simulink model "Ex1Mdl"  (R2019b)
settings: Solver=VariableStepAuto  StartTime=0.0  StopTime=20  RelTol=1e-3
values from neighbouring files (symbols this model uses):
  k1 = p(4)    [Ex1.m]
  k2 = p(3)    [Ex1.m]
  k3 = p(2)    [Ex1.m]
  z0 = [0.001 0 0.2]    [Ex1.m]
settings Model: Creator=Administrator  LastModifiedBy=jiachenqin
settings DataIOCC: SaveOutput=off  SignalLogging=off  DSMLogging=off  SaveTime=off  ReturnWorkspaceOutputs=off
settings SFSimCC: CustomCodeUndefinedFunction=UseInterfaceOnly

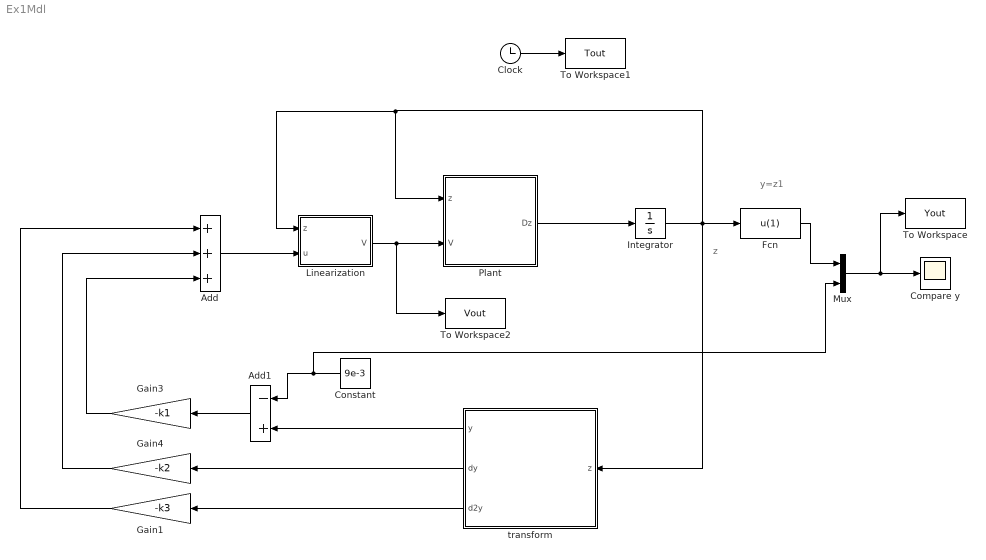
== system Ex1Mdl ==
  note: z
  note: y=z1
  Add : Sum  Inputs=+++
  Add1 : Sum  Inputs=-+
  Clock : Clock
  Compare y : Scope
  Constant : Constant  Value=9e-3
  Fcn : Fcn  Expr=u(1)
  Gain1 : Gain  Gain=-k3
  Gain3 : Gain  Gain=-k1
  Gain4 : Gain  Gain=-k2
  Integrator : Integrator  InitialCondition=z0
  Linearization : MATLAB Function  TreatAsAtomicUnit=on
  Mux : Mux  Inputs=2
  Plant : MATLAB Function  TreatAsAtomicUnit=on
  To Workspace : ToWorkspace  VariableName=Yout  SampleTime=-1
  To Workspace1 : ToWorkspace  VariableName=Tout  SampleTime=-1
  To Workspace2 : ToWorkspace  VariableName=Vout  SampleTime=-1
  transform : MATLAB Function  TreatAsAtomicUnit=on
  wires:
  Integrator/1 -> transform/1(z), Fcn/1, Linearization/1(z), Plant/1(z)
  Plant/1(Dz) -> Integrator/1
  Linearization/1(V) -> To Workspace2/1, Plant/2(V)
  Add/1 -> Linearization/2(u)
  transform/1(y) -> Add1/2
  transform/2(dy) -> Gain4/1
  transform/3(d2y) -> Gain1/1
  Constant/1 -> Mux/2, Add1/1
  Add1/1 -> Gain3/1
  Gain3/1 -> Add/3
  Gain4/1 -> Add/2
  Gain1/1 -> Add/1
  Fcn/1 -> Mux/1
  Mux/1 -> To Workspace/1, Compare y/1
  Clock/1 -> To Workspace1/1

== matlab function Ex1Mdl/Linearization ==
  data: z input; V output; u input
function V = fcn(z,u)

z1 = z(1);
z2 = z(2);
z3 = z(3);

% Paramerters
L = 0.4125;
R1 = 10;
Rs = 1;
G = 3.2654e-5;
m = 0.068;
g = 9.8;

Lf3hz = (2*G*z2*z3^2)/(m*z1^3) + (2*G*z3^2*(R1 + Rs))/(L*m*z1^2);
LgLf2hz = -(2*G*z3)/(L*m*z1^2);

V = (u  - Lf3hz) / LgLf2hz;

== matlab function Ex1Mdl/Plant ==
  data: z input; Dz output; V input
function Dz = fcn(z,V)

% Paramerters
L = 0.4125;
R1 = 10;
Rs = 1;
G = 3.2654e-5;
m = 0.068;
g = 9.8;

z1 = z(1);
z2 = z(2);
z3 = z(3);


Dz = [z2; g-G*z3^2/(m*z1^2); V/L-(R1+Rs)*z3/L ];

== matlab function Ex1Mdl/transform ==
  data: z input size=3; y output; dy output; d2y output
function [y,dy,d2y] = fcn(z)

z1 = z(1);
z2 = z(2);
z3 = z(3);


% Paramerters
L = 0.4125;
R1 = 10;
Rs = 1;
G = 3.2654e-5;
m = 0.068;
g = 9.8;

y = z1;
dy = z2;
d2y = g-G*z3^2/(m*z1^2);
